simulink model "VSG_Test"  (R2022b)
settings: Solver=VariableStepAuto  StartTime=0.0  StopTime=10.0  RelTol=1e-3
settings Model: Creator=TKWTL  LastModifiedBy=TKWTL

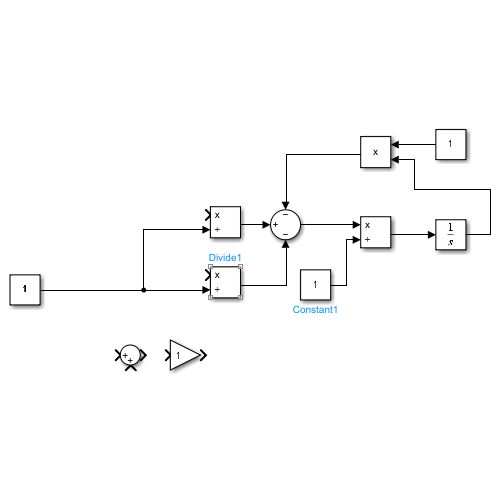
[thumbnail: Simulink's stored preview of the top-level diagram]
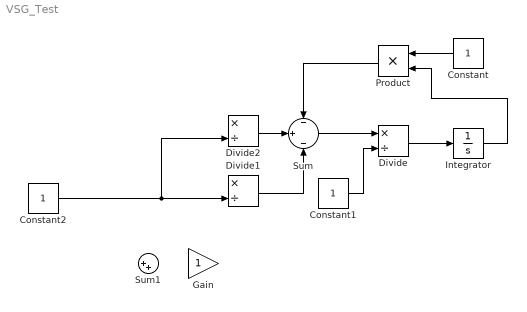
== system VSG_Test ==
  Constant : Constant
  Constant1 : Constant
  Constant2 : Constant
  Divide : Product  Inputs=*/
  Divide1 : Product  Inputs=*/
  Divide2 : Product  Inputs=*/
  Gain : Gain
  Integrator : Integrator
  Product : Product
  Sum : Sum  Inputs=-|+|-
  Sum1 : Sum  Inputs=|++
  wires:
  Divide/1 -> Integrator/1
  Sum/1 -> Divide/1
  Divide1/1 -> Sum/3
  Constant1/1 -> Divide/2
  Constant/1 -> Product/1
  Integrator/1 -> Product/2
  Product/1 -> Sum/1
  Divide2/1 -> Sum/2
  Constant2/1 -> Divide2/2, Divide1/2
